simulink model "TPS_failure_systemV20"  (R2020a)
settings: Solver=FixedStepDiscrete  StartTime=0.0  StopTime=10.0  FixedStep=.1  RelTol=1e-3
libraries: simulink x5
settings Model: Creator=Administrator  LastModifiedBy=Administrator
settings OptimizationCC: DefaultParameterBehavior=Inlined  EnhancedBackFolding=on  PassReuseOutputArgsAs=Individual arguments  ZeroExternalMemoryAtStartup=off  ZeroInternalMemoryAtStartup=off  OptimizeBlockOrder=speed  DifferentSizesBufferReuse=on  OptimizationCustomize=off  EfficientTunableParamExpr=on
settings DebuggingCC: ParameterTunabilityLossMsg=error  UnconnectedInputMsg=none  UnconnectedOutputMsg=none  UnconnectedLineMsg=none
settings HardwareCC: ProdBitPerPointer=32  ProdBitPerSizeT=32  ProdBitPerPtrDiffT=32  ProdLargestAtomicInteger=Long  ProdLargestAtomicFloat=Double  ProdWordSize=32  ProdHWDeviceType=ARM Compatible->ARM Cortex
settings ModelReferenceCC: EnableRefExpFcnMdlSchedulingChecks=off
settings SFSimCC: MATLABDynamicMemAlloc=off
settings RTWCC: SystemTargetFile=ert.tlc  GenCodeOnly=on  TemplateMakefile=ert_default_tmf
settings CodeAppCC: ForceParamTrailComments=on  IgnoreCustomStorageClasses=off  OperatorAnnotations=on  SimulinkDataObjDesc=on  SFDataObjDesc=on  InsertBlockDesc=on
settings ERTTargetCC: TargetLangStandard=C99 (ISO)  GenerateSampleERTMain=on  InlinedParameterPlacement=NonHierarchical  ERTCustomFileTemplate=example_file_process.tlc

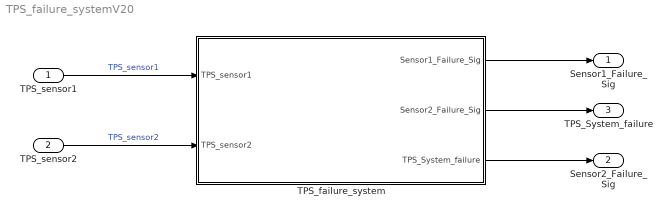
== system TPS_failure_systemV20 ==
  TPS_sensor1 : Inport  OutDataTypeStr=single
  TPS_sensor2 : Inport  Port=2  OutDataTypeStr=single
  TPS_failure_system : Subsystem
  Sensor1_Failure_Sig : Outport  OutDataTypeStr=boolean
  Sensor2_Failure_Sig : Outport  Port=2  OutDataTypeStr=boolean
  TPS_System_failure : Outport  Port=3  OutDataTypeStr=boolean
  wires:
  TPS_failure_system/1(Sensor1_Failure_Sig) -> Sensor1_Failure_Sig/1
  TPS_failure_system/2(Sensor2_Failure_Sig) -> TPS_System_failure/1
  TPS_failure_system/3(TPS_System_failure) -> Sensor2_Failure_Sig/1
  TPS_sensor1/1 -> TPS_failure_system/1(TPS_sensor1)  "TPS_sensor1"
  TPS_sensor2/1 -> TPS_failure_system/2(TPS_sensor2)  "TPS_sensor2"

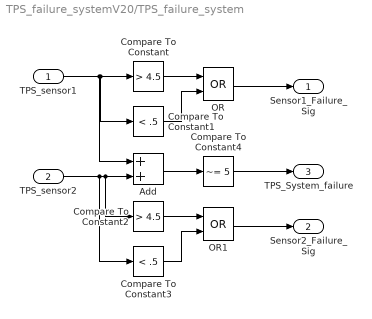
== system TPS_failure_systemV20/TPS_failure_system ==
  TPS_sensor1 : Inport  OutDataTypeStr=single
  TPS_sensor2 : Inport  Port=2  OutDataTypeStr=single
  Add : Sum
  Compare To Constant : simulink/Logic and Bit Operations/Compare To Constant  relop=>  const=4.5  OutDataTypeStr=boolean
  Compare To Constant1 : simulink/Logic and Bit Operations/Compare To Constant  relop=<  const=.5  OutDataTypeStr=boolean
  Compare To Constant2 : simulink/Logic and Bit Operations/Compare To Constant  relop=>  const=4.5  OutDataTypeStr=boolean
  Compare To Constant3 : simulink/Logic and Bit Operations/Compare To Constant  relop=<  const=.5  OutDataTypeStr=boolean
  Compare To Constant4 : simulink/Logic and Bit Operations/Compare To Constant  relop=~=  const=5  OutDataTypeStr=boolean
  OR : Logic  Operator=OR  AllPortsSameDT=off  OutDataTypeStr=boolean
  OR1 : Logic  Operator=OR  AllPortsSameDT=off  OutDataTypeStr=boolean
  Sensor1_Failure_Sig : Outport  OutDataTypeStr=boolean
  Sensor2_Failure_Sig : Outport  Port=2  OutDataTypeStr=boolean
  TPS_System_failure : Outport  Port=3  OutDataTypeStr=boolean
  wires:
  TPS_sensor2/1 -> Add/2, Compare To Constant2/1, Compare To Constant3/1
  TPS_sensor1/1 -> Compare To Constant1/1, Compare To Constant/1, Add/1
  OR/1 -> Sensor1_Failure_Sig/1
  Compare To Constant/1 -> OR/1
  Compare To Constant2/1 -> OR1/1
  Compare To Constant1/1 -> OR/2
  Compare To Constant4/1 -> TPS_System_failure/1
  Compare To Constant3/1 -> OR1/2
  Add/1 -> Compare To Constant4/1
  OR1/1 -> Sensor2_Failure_Sig/1
